simulink model "bluetooth_voice_article"  (Simulink 4.00)
settings: Solver=VariableStepDiscrete  StartTime=0.0  StopTime=2.7  RelTol=1e-3
PreLoadFcn:
  | bluetooth_init;
StopFcn:
  | ratio=sum((hops>=29) & (hops<=49))/length(hops)
values from neighbouring files (symbols this model uses):
  Access_Code = zeros(72,1); Access_Code(1:2:72)=1    [bluetooth_init.m]
  ARQ = [1]    [bluetooth_init.m]
  awgn_channel_seed = randseed(2)    [bluetooth_init.m]
  Flow_Control = [1]    [bluetooth_init.m]
  Input_Fs = 8000    [bluetooth_init.m]
  One_Zero_Payload = zeros(240,1)    [bluetooth_init.m]
  Packet_Type = [1 0 1 0]'    [bluetooth_init.m]
  Sequence = [1]    [bluetooth_init.m]
  Slave_Address = [1 0 1]'    [bluetooth_init.m]
undefined symbols (not defined in the file or in its folder): Fs, g, jet
libraries: dspsrcs3 x20, dspsigops x11, simulink3 x10, dspsigattribs x8, bluetooth_lib x5, dspmathops x4, dspbuff3 x4, dspsnks3 x4, commsink2 x3, dspmtrx3 x3, commdigbbndfm2 x3, dspindex x2
Description:
  | Bluetooth Voice Model
  | 
  | Associated Files:
  | bluetooth_init.m: Initialization
  | bluetooth_lib.mdl: Library
  | poiss_gaus_prc3.m: Poisson S-function for 802.11
  | scomdemohecgen.c: S-function C code for CRC block
  | scomdemohecgen.dll: S-function dll for CRC block
  | input.wav: Input wave file
settings Model: Creator=Stuart McGarrity  LastModifiedBy=stuartm  SaveTime=off  SaveOutput=off  OptimizeBlockIOStorage=off  BlockReductionOpt=off
settings Model: ModifiedComment=|
  | stuartm -- Fri Jul 20 12:58:27 2001 -- Version 1.201
  | Fix for R12.1. Changed CPM modulator. Replaced enable subsystems in channel with "switch case".
settings Model: ModifiedHistory=|
  | stuartm -- Fri Jul 20 12:58:27 2001 -- Version 1.201
  | Fix for R12.1. Changed CPM modulator. Replaced enable subsystems in channel with "switch case".
  | 
  | 
  | stuartm -- Sun Jul 08 13:59:13 2001 -- Version 1.172
  | Added gain mask at output of transmitter to run it off after 374 bits.
  | 
  | stuartm -- Sun Jul 08 13:53:19 2001 -- Version 1.171
  | Changed hop generator to randint block. Put zero padiing back to before transmitter.
  | 
  | 
  | Started with bluetooth_voice2. Move zero pad from input to output of transmitter. Now only transmits 374 bits
  | 
  | Added channel option

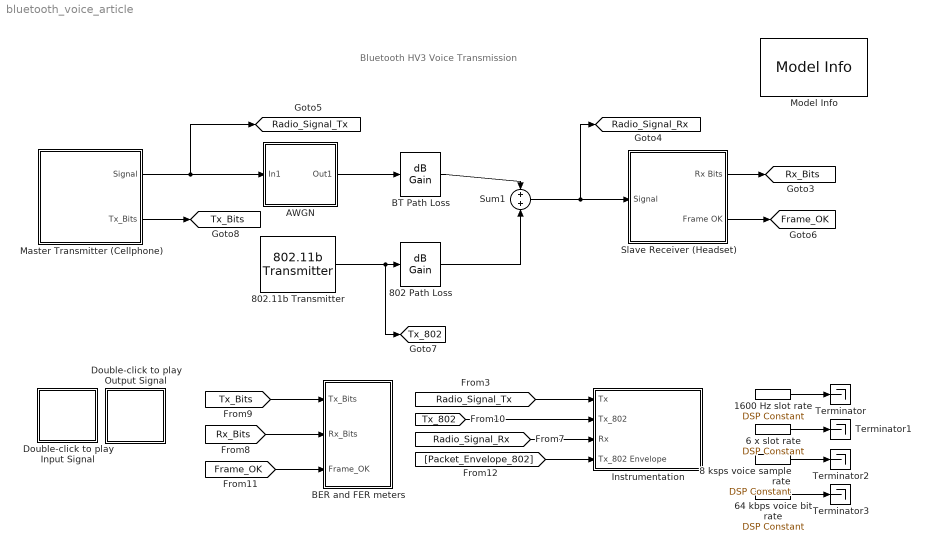
== system bluetooth_voice_article ==
  note: Bluetooth
      |  HV3 Voice Transmission
  1600 Hz slot rate : dspsrcs3/DSP Constant  Value=1  InterpretAs1D=off  SampleMode=Discrete  Ts=1/1600  FramebasedOutput=off
  6 x slot rate : dspsrcs3/DSP Constant  Value=1  InterpretAs1D=off  SampleMode=Discrete  Ts=6/1600  FramebasedOutput=off
  64 kbps voice bit rate : dspsrcs3/DSP Constant  Value=1  InterpretAs1D=off  SampleMode=Discrete  Ts=1/64000  FramebasedOutput=off
  8 ksps voice sample rate : dspsrcs3/DSP Constant  Value=1  InterpretAs1D=off  SampleMode=Discrete  Ts=1/8000  FramebasedOutput=off
  802 Path Loss : dspmathops/dB Gain  Gain=g  dB=-40  intype=Amplitude
  802.11b Transmitter : bluetooth_lib/802.11b Transmitter  On=on  rate=200  m=1e-3  v=0  power=1  Freq_Number=39  rate_seed=rate_802_seed  awgn_seed=awgn_802_seed
  AWGN : Subsystem  TreatAsAtomicUnit=on  mask(Optional channel){AWGN_On=on, EsNo=5, Power=.001, Symbol_Period=1e-6, seed=awgn_channel_seed}
      mask prompts: AWGN_On "Turn on AWGN"; EsNo "Es/No"; Power "Input Power"; Symbol_Period "Symbol Period"
      mask init:
      | if AWGN_On==1
      |    Name='On';
      | else
      |   Name='Off';
      | end;
      settings: RTWFcnNameOpts=Auto  RTWFileNameOpts=Auto
      mask Display: disp(['AWGN is ' Name])
  BER and FER meters : Subsystem
      settings: RTWFcnNameOpts=Auto  RTWFileNameOpts=Auto
  BT Path Loss : dspmathops/dB Gain  Gain=g  dB=-40  intype=Amplitude
  Double-click to play Input Signal : Subsystem  mask(Plot histogram){}
      mask init:
      | [x,y,x1,y1,x2,y2] = dspblkwao2('icon');
      settings: OpenFcn=[Input_Wave,Input_Fs]=wavread('Input.wav');sound(Input_Wave,Input_Fs);  RTWFcnNameOpts=Auto  RTWFileNameOpts=Auto
      mask Display:
      | patch(x1,y1,[1 1 1]*.5);
      | patch(x2,y2);
      | plot(x,y); plot(x1,y1)
  Double-click to play Output Signal : Subsystem  mask(Plot histogram){}
      mask init:
      | [x,y,x1,y1,x2,y2] = dspblkwao2('icon');
      settings: OpenFcn=[Output_Wave,Output_Fs]=wavread('Output.wav');sound(Output_Wave,Output_Fs);  RTWFcnNameOpts=Auto  RTWFileNameOpts=Auto
      mask Display:
      | patch(x1,y1,[1 1 1]*.5);
      | patch(x2,y2);
      | plot(x,y); plot(x1,y1)
  Instrumentation : Subsystem  TreatAsAtomicUnit=on  mask(Instrumentation){On=on, Off=off}
      mask init:
      | if strcmp(On,'on')
      |   string='Instrumentation\nis On\n(Double-Click\n to Toggle)\n ';
      |   set_param([gcb,'/State'],'Value','1');
      | else
      |   string='Instrumentation\nis Off\n(Double-Click\n to Toggle)\n ';
      |   set_param([gcb,'/State'],'Value','0');
      | end
      settings: OpenFcn=temp=get_param(gcb,'On');set_param(gcb,'On', get_param(gcb,'Off'));set_param(gcb,'Off', temp);  RTWFcnNameOpts=Auto  RTWFileNameOpts=Auto
      mask Display: disp(string);
  Master Transmitter (Cellphone) : Subsystem
      settings: RTWFcnNameOpts=Auto  RTWFileNameOpts=Auto
      mask Display: plot(0,0,100,100,[30,60,60,55,55,30,30],[10,10,90,90,70,70,10],[35,35,55,55,35],[64,45,45,64,64])
  Model Info : simulink3/Signals & Systems/Model Info  InitialBlockCM=none  BlockCM=none  Frame=on  DisplayStringWithTags=|  HorizontalTextAlignment=Center  LeftAlignmentValue=0.5  SourceBlockDiagram=bluetooth_voice  TagMaxNumber=20
      | Bluetooth Voice
      | %<ModelVersion>
  Slave Receiver (Headset) : Subsystem
      settings: RTWFcnNameOpts=Auto  RTWFileNameOpts=Auto
      mask Display: plot(15,5,95,80,[26, 28,35,44,58,85,87,92,86,59,46,46,38, 31, 27,26],[55,49,45,45,34,15,10,16,17,37,50,58,66,67,62,55],[32,34,37,42,46,46],[67,69,71,70,66,58],[27,25,24,21,23,26],[52,49,45,47,52,58],[35,38,40,42,44],[66,67,66,64,61],[34,32,38,40,34],[60,56,51,55,60])
  Sum1 : Sum  Inputs=++  SaturateOnIntegerOverflow=on
  Terminator{,1..3} (4 alike) : Terminator
  tag scope: Frame_OK=global, Radio_Signal_Rx=global, Radio_Signal_Tx=global, Rx_Bits=global, Tx_802=global, Tx_Bits=global
  wires:
  Master Transmitter (Cellphone)/1(Signal) -> [Radio_Signal_Tx], AWGN/1(In1)
  [Radio_Signal_Tx] -> Instrumentation/1(Tx)
  [Radio_Signal_Rx] -> Instrumentation/3(Rx)
  [Frame_OK] -> BER and FER meters/3(Frame_OK)
  [Tx_Bits] -> BER and FER meters/1(Tx_Bits)
  [Rx_Bits] -> BER and FER meters/2(Rx_Bits)
  [Tx_802] -> Instrumentation/2(Tx_802)
  [Packet_Envelope_802] -> Instrumentation/4(Tx_802 Envelope)
  802.11b Transmitter/1 -> [Tx_802], 802 Path Loss/1
  AWGN/1(Out1) -> BT Path Loss/1
  BT Path Loss/1 -> Sum1/1
  Sum1/1 -> [Radio_Signal_Rx], Slave Receiver (Headset)/1(Signal)
  802 Path Loss/1 -> Sum1/2
  Master Transmitter (Cellphone)/2(Tx_Bits) -> [Tx_Bits]
  Slave Receiver (Headset)/1(Rx Bits) -> [Rx_Bits]
  Slave Receiver (Headset)/2(Frame OK) -> [Frame_OK]
  1600 Hz slot rate/1 -> Terminator/1
  6 x slot rate/1 -> Terminator1/1
  8 ksps voice sample rate/1 -> Terminator2/1
  64 kbps voice bit rate/1 -> Terminator3/1

== system bluetooth_voice_article/AWGN ==
  In1 : Inport  Port=1  LatchInput=off
  Generate noise only for slot 1 : simulink3/Nonlinear/Manual Switch  sw=0  action=0
  Mode : Constant  Value=AWGN_On
  Slot 1 enable2 : dspsrcs3/Signal From Workspace  X=[1 0 0 0 0 0]  Ts=625e-6  nsamps=1  OutputAfterFinalValue=Cyclic Repetition
  Slot 1 enable3 : dspsrcs3/Signal From Workspace  X=[1 1 1 1 1 1 ]  Ts=625e-6  nsamps=1  OutputAfterFinalValue=Cyclic Repetition
  Subsystem : Subsystem  TreatAsAtomicUnit=on
      settings: RTWFcnNameOpts=Auto  RTWFileNameOpts=Auto
  Out1 : Outport  Port=1  InitialOutput=0
  wires:
  Mode/1 -> Subsystem/1(In1)
  Subsystem/1(Out1) -> Out1/1
  Slot 1 enable3/1 -> Generate noise only for slot 1/2
  Generate noise only for slot 1/1 -> Subsystem/Enable
  Slot 1 enable2/1 -> Generate noise only for slot 1/1
  In1/1 -> Subsystem/2(In2)

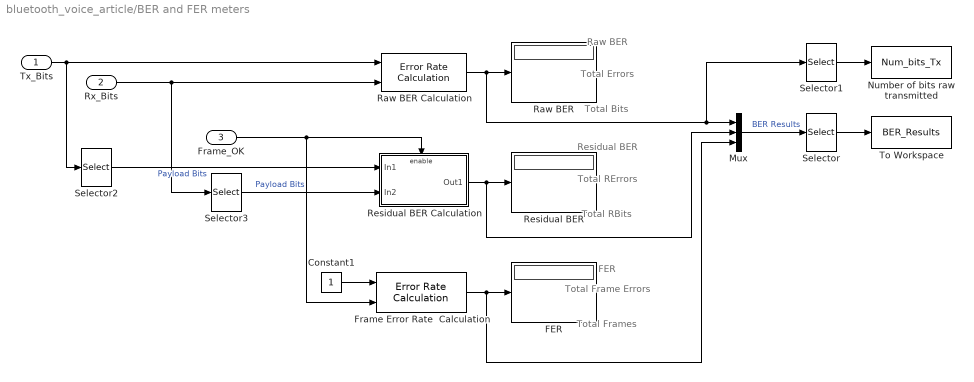
== system bluetooth_voice_article/BER and FER meters ==
  note: Residual BER
  note: Total RBits
  note: Total RErrors
  note: FER
  note: Total Frames
  note: Total Frame Errors
  note: Raw BER
  note: Total Bits
  note: Total Errors
  Tx_Bits : Inport  Port=1  LatchInput=off
  Rx_Bits : Inport  Port=2  LatchInput=off
  Frame_OK : Inport  Port=3  LatchInput=off
  Constant1 : Constant  Value=1
  FER : Display
      settings: Format=short
  Frame Error Rate  Calculation : commsink2/Error Rate Calculation  N=0  st_delay=0  cp_mode=Entire frame  subframe=[]  PMode=Port  WsName=ErrorVec  RsMode2=off  stop=off  numErr=100  maxBits=1e6
  Mux : Mux  Inputs=3
  Number of bits raw transmitted : ToWorkspace  VariableName=Num_bits_Tx  SampleTime=-1  SaveFormat=Array
      settings: MaxDataPoints=1
  Raw BER : Display
      settings: Format=short
  Raw BER Calculation : commsink2/Error Rate Calculation  N=0  st_delay=0  cp_mode=Entire frame  subframe=[]  PMode=Port  WsName=ErrorVec  RsMode2=off  stop=off  numErr=100  maxBits=1e6
  Residual BER : Display
      settings: Format=short
  Residual BER Calculation : Subsystem  TreatAsAtomicUnit=on
      settings: RTWFcnNameOpts=Auto  RTWFileNameOpts=Auto
  Selector : Selector  InputType=Vector  ElementSrc=Internal  Elements=[1 4 7]  RowSrc=Internal  Rows=1  ColumnSrc=Internal  Columns=1  InputPortWidth=9
  Selector1 : Selector  InputType=Vector  ElementSrc=Internal  Elements=[3]  RowSrc=Internal  Rows=1  ColumnSrc=Internal  Columns=1  InputPortWidth=3
  Selector2 : Selector  InputType=Vector  ElementSrc=Internal  Elements=[127:366]  RowSrc=Internal  Rows=1  ColumnSrc=Internal  Columns=1  InputPortWidth=366
  Selector3 : Selector  InputType=Vector  ElementSrc=Internal  Elements=[127:366]  RowSrc=Internal  Rows=1  ColumnSrc=Internal  Columns=1  InputPortWidth=366
  To Workspace : ToWorkspace  VariableName=BER_Results  SampleTime=-1  SaveFormat=Array
      settings: MaxDataPoints=1
  wires:
  Residual BER Calculation/1(Out1) -> Residual BER/1, Mux/2
  Frame_OK/1 -> Residual BER Calculation/Enable, Frame Error Rate  Calculation/2
  Frame Error Rate  Calculation/1 -> FER/1, Mux/3
  Tx_Bits/1 -> Raw BER Calculation/1, Selector2/1
  Rx_Bits/1 -> Raw BER Calculation/2, Selector3/1
  Raw BER Calculation/1 -> Raw BER/1, Mux/1, Selector1/1
  Mux/1 -> Selector/1  "BER Results"
  Selector/1 -> To Workspace/1
  Constant1/1 -> Frame Error Rate  Calculation/1
  Selector1/1 -> Number of bits raw transmitted/1
  Selector3/1 -> Residual BER Calculation/2(In2)  "Payload Bits"
  Selector2/1 -> Residual BER Calculation/1(In1)  "Payload Bits"

== system bluetooth_voice_article/Double-click to play Input Signal ==

== system bluetooth_voice_article/Double-click to play Output Signal ==

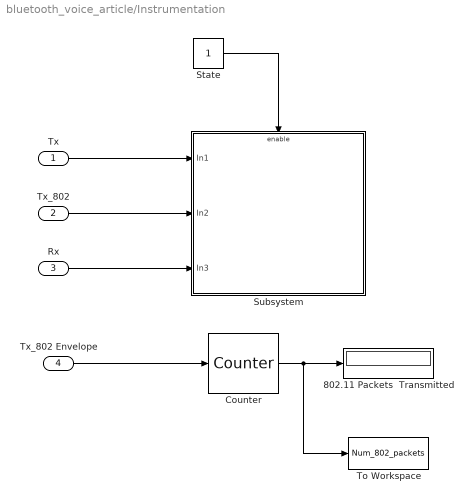
== system bluetooth_voice_article/Instrumentation ==
  Tx : Inport  Port=1  LatchInput=off
  Tx_802 : Inport  Port=2  LatchInput=off
  Rx : Inport  Port=3  LatchInput=off
  Tx_802 Envelope : Inport  Port=4  LatchInput=off
  802.11 Packets  Transmitted : Display
      settings: Format=short
  Counter : dspswit3/Counter  Direction=Up  CountEvent=Rising edge  CounterSize=User defined  MaxCount=1000  InitialCount=0  Output=Count  HitValue=32  ResetInput=off  SamplesPerFrame=1  Ts=1
  State : Constant  Value=1
  Subsystem : Subsystem  TreatAsAtomicUnit=on
      settings: RTWFcnNameOpts=Auto  RTWFileNameOpts=Auto
  To Workspace : ToWorkspace  VariableName=Num_802_packets  SampleTime=-1  SaveFormat=Array
      settings: MaxDataPoints=1
  wires:
  Rx/1 -> Subsystem/3(In3)
  Tx/1 -> Subsystem/1(In1)
  Tx_802/1 -> Subsystem/2(In2)
  Tx_802 Envelope/1 -> Counter/1
  State/1 -> Subsystem/Enable
  Counter/1 -> 802.11 Packets  Transmitted/1, To Workspace/1

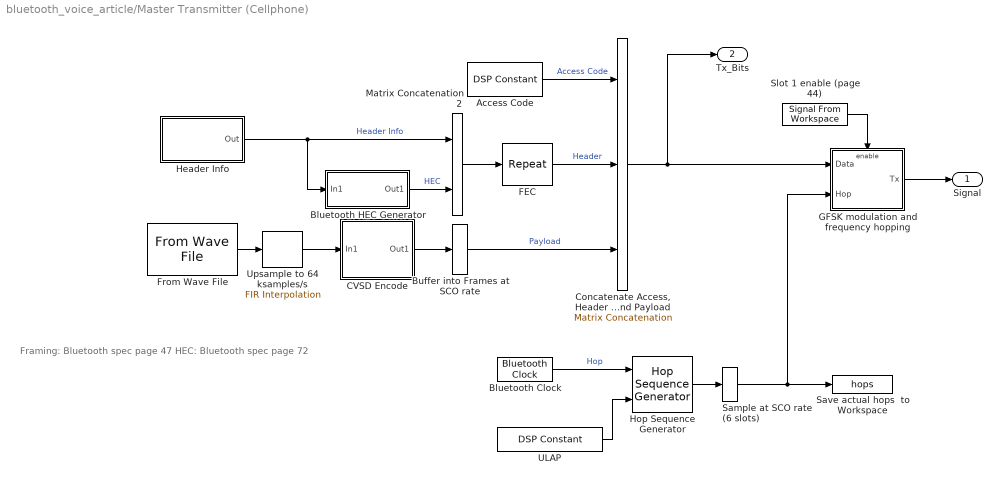
== system bluetooth_voice_article/Master Transmitter (Cellphone) ==
  note: Framing: Bluetooth spec page 47
      | HEC: Bluetooth spec page 72
  Access Code : dspsrcs3/DSP Constant  Value=Access_Code  InterpretAs1D=off  SampleMode=Discrete  Ts=30*(1/Input_Fs)  FramebasedOutput=on
  Bluetooth Clock : bluetooth_lib/Bluetooth Clock  Ts=(1/1600)/2
  Bluetooth HEC Generator : Subsystem  mask(Bluetooth HEC Generator){uap=[1 0 0 1 0 1 1 0]}
      mask help: Compute the Bluetooth Header Error Check (HEC) as specified in section 5.4 of the Bluetooth specification. The Upper Address Part (UAP) is used to initialize the state of the encoder. The UAP is an 8-bit vector, LSB first.
      settings: RTWFcnNameOpts=Auto  RTWFileNameOpts=Auto
      mask Display: disp('Bluetooth\nHEC Generator')
  Buffer into Frames at SCO rate : dspbuff3/Buffer  N=240  V=0  ic=One_Zero_Payload
  CVSD Encode : Subsystem  mask(CVSD Encoder){min_step=10, max_step=1280, accum_decay=1-1/32, step_decay=1-1/1024}
      mask prompts: min_step "Minimum Step Size"; max_step "Maximum Step Size"; accum_decay "Accumulator Decay"; step_decay "Step Decay"
      mask help: Encode a 64 K samples per sec speech signal into a 64Kbps bit stream.
      mask init:
      | pos_accum_max = 2^15 - 1;
      | neg_accum_max = -2^15 + 1;
      settings: RTWFcnNameOpts=Auto  RTWFileNameOpts=Auto
      mask Display: disp('CVSD\nEncode')
  "Concatenate Access, Header and Payload" : simulink3/Signals & Systems/Matrix Concatenation  numInports=3  catMethod=Vertical
  FEC : dspsigops/Repeat  N=3  ic=0  mode=Maintain input frame rate
  From Wave File : dspsrcs3/From Wave File  FileName=Input.wav  SamplesPerFrame=1  MinBufSize=256
  GFSK modulation and frequency hopping : Subsystem  TreatAsAtomicUnit=on
      settings: RTWFcnNameOpts=Auto  RTWFileNameOpts=Auto
  Header Info : Subsystem
      settings: RTWFcnNameOpts=Auto  RTWFileNameOpts=Auto
      mask Display: disp('Header Info')
  Hop Sequence Generator : bluetooth_lib/Hop Sequence Generator  Hop_Mode=Connection State Hop Sequence  hop_seed=hop_seed  fixed_hop_freq=fixed_hop_freq
  Matrix Concatenation2 : simulink3/Signals & Systems/Matrix Concatenation  numInports=2  catMethod=Vertical
  Sample at SCO rate (6 slots) : ZeroOrderHold  SampleTime=6*625e-6
  Save actual hops  to Workspace : ToWorkspace  VariableName=hops  SampleTime=-1  SaveFormat=Array
  Slot 1 enable (page 44) : dspsrcs3/Signal From Workspace  X=[1 0 0 0 0 0]  Ts=625e-6  nsamps=1  OutputAfterFinalValue=Cyclic Repetition
  ULAP : dspsrcs3/DSP Constant  Value=hex2dec('2a96ef25')  InterpretAs1D=off  SampleMode=Discrete  Ts=(1/1600)/2  FramebasedOutput=off
  Upsample to 64 ksamples/s : dspmlti3/FIR Interpolation  h=interp_coeffs  L=8  framing=Maintain input frame size  outputBufInitCond=0
  Signal : Outport  Port=1
  Tx_Bits : Outport  Port=2
  wires:
  Slot 1 enable (page 44)/1 -> GFSK modulation and frequency hopping/Enable
  GFSK modulation and frequency hopping/1(Tx) -> Signal/1
  CVSD Encode/1(Out1) -> Buffer into Frames at SCO rate/1
  From Wave File/1 -> Upsample to 64 ksamples/s/1
  Upsample to 64 ksamples/s/1 -> CVSD Encode/1(In1)
  Buffer into Frames at SCO rate/1 -> "Concatenate Access, Header and Payload"/3  "Payload"
  Access Code/1 -> "Concatenate Access, Header and Payload"/1  "Access Code"
  "Concatenate Access, Header and Payload"/1 -> Tx_Bits/1, GFSK modulation and frequency hopping/1(Data)
  FEC/1 -> "Concatenate Access, Header and Payload"/2  "Header"
  Header Info/1(Out) -> Bluetooth HEC Generator/1(In1), Matrix Concatenation2/1  "Header Info"
  Bluetooth HEC Generator/1(Out1) -> Matrix Concatenation2/2  "HEC"
  Matrix Concatenation2/1 -> FEC/1
  Hop Sequence Generator/1 -> Sample at SCO rate (6 slots)/1
  ULAP/1 -> Hop Sequence Generator/2
  Sample at SCO rate (6 slots)/1 -> GFSK modulation and frequency hopping/2(Hop), Save actual hops  to Workspace/1
  Bluetooth Clock/1 -> Hop Sequence Generator/1  "Hop"

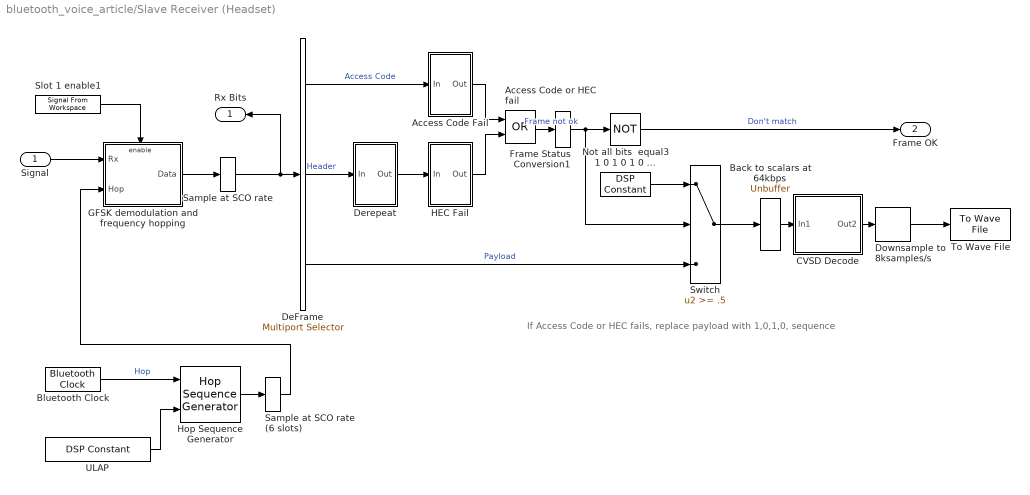
== system bluetooth_voice_article/Slave Receiver (Headset) ==
  note: If Access Code or HEC fails,
      | replace payload with 1,0,1,0, sequence
  Signal : Inport  Port=1  LatchInput=off
  1 0 1 0 1 0 ... : dspsrcs3/DSP Constant  Value=One_Zero_Payload  InterpretAs1D=off  SampleMode=Discrete  Ts=30*(1/Input_Fs)  FramebasedOutput=on
  Access Code Fail : Subsystem
      settings: RTWFcnNameOpts=Auto  RTWFileNameOpts=Auto
  Access Code or HEC fail : Logic  Operator=OR  Inputs=2
  Back to scalars at 64kbps : dspbuff3/Unbuffer  ic=0
  Bluetooth Clock : bluetooth_lib/Bluetooth Clock  Ts=(1/1600)/2
  CVSD Decode : Subsystem  TreatAsAtomicUnit=on  mask(CVSD Decoder){min_step=10, max_step=1280, accum_decay=1-1/32, step_decay=1-1/1024}
      mask prompts: min_step "Minimum Step Size"; max_step "Maximum Step Size"; accum_decay "Accumulator Decay"; step_decay "Step Decay"
      mask init:
      | pos_accum_max = 2^15 - 1;
      | neg_accum_max = -2^15 + 1;
      settings: RTWFcnNameOpts=Auto  RTWFileNameOpts=Auto
      mask Display: disp('CVSD\nDecoder')
  DeFrame : dspindex/Multiport Selector  rowsOrCols=Rows  idxCellArray={ 1:72, 73:126,127:366}  idxErrMode=Clip Index
  Derepeat : Subsystem
      settings: RTWFcnNameOpts=Auto  RTWFileNameOpts=Auto
  Downsample to 8ksamples/s : dspsigops/Downsample  N=8  phase=0  ic=0  smode=Allow multirate  fmode=Maintain input frame size
  Frame Status Conversion1 : dspsigattribs/Frame Status Conversion  growRefPort=off  outframe=Sample-based
  GFSK demodulation and frequency hopping : Subsystem  TreatAsAtomicUnit=on
      settings: RTWFcnNameOpts=Auto  RTWFileNameOpts=Auto
  HEC Fail : Subsystem
      settings: RTWFcnNameOpts=Auto  RTWFileNameOpts=Auto
  Hop Sequence Generator : bluetooth_lib/Hop Sequence Generator  Hop_Mode=Connection State Hop Sequence  hop_seed=hop_seed  fixed_hop_freq=fixed_hop_freq
  Not all bits  equal3 : Logic  Operator=NOT  Inputs=1
  Sample at SCO rate : ZeroOrderHold  SampleTime=6*625e-6
  Sample at SCO rate (6 slots) : ZeroOrderHold  SampleTime=6*625e-6
  Slot 1 enable1 : dspsrcs3/Signal From Workspace  X=[1 0 0 0 0 0]  Ts=625e-6  nsamps=1  OutputAfterFinalValue=Cyclic Repetition
  Switch : Switch  Threshold=.5
  To Wave File : dspsnks3/To Wave File  filename=Output  sampleWidth=8  MinNumSamples=256
  ULAP : dspsrcs3/DSP Constant  Value=hex2dec('2a96ef25')  InterpretAs1D=off  SampleMode=Discrete  Ts=(1/1600)/2  FramebasedOutput=off
  Rx Bits : Outport  Orientation=left  Port=1
  Frame OK : Outport  Port=2
  wires:
  GFSK demodulation and frequency hopping/1(Data) -> Sample at SCO rate/1
  Slot 1 enable1/1 -> GFSK demodulation and frequency hopping/Enable
  Signal/1 -> GFSK demodulation and frequency hopping/1(Rx)
  Not all bits  equal3/1 -> Frame OK/1  "Don't match"
  CVSD Decode/1(Out2) -> Downsample to 8ksamples/s/1
  Downsample to 8ksamples/s/1 -> To Wave File/1
  Back to scalars at 64kbps/1 -> CVSD Decode/1(In1)
  Sample at SCO rate/1 -> DeFrame/1, Rx Bits/1
  Sample at SCO rate (6 slots)/1 -> GFSK demodulation and frequency hopping/2(Hop)
  DeFrame/2 -> Derepeat/1(In)  "Header"
  DeFrame/3 -> Switch/3  "Payload"
  DeFrame/1 -> Access Code Fail/1(In)  "Access Code"
  Access Code or HEC fail/1 -> Frame Status Conversion1/1  "Frame not ok"
  1 0 1 0 1 0 .../1 -> Switch/1
  Access Code Fail/1(Out) -> Access Code or HEC fail/1
  Derepeat/1(Out) -> HEC Fail/1(In)
  HEC Fail/1(Out) -> Access Code or HEC fail/2
  Frame Status Conversion1/1 -> Switch/2, Not all bits  equal3/1
  Switch/1 -> Back to scalars at 64kbps/1
  Hop Sequence Generator/1 -> Sample at SCO rate (6 slots)/1
  ULAP/1 -> Hop Sequence Generator/2
  Bluetooth Clock/1 -> Hop Sequence Generator/1  "Hop"

== system bluetooth_voice_article/AWGN/Subsystem ==
  In1 : Inport  Port=1  LatchInput=off
  In2 : Inport  Port=2  LatchInput=off
  Enable : EnablePort
  Add noise : Subsystem  TreatAsAtomicUnit=on
      settings: RTWFcnNameOpts=Auto  RTWFileNameOpts=Auto
  If : If  NumInputs=1  IfExpression=u1 == 0  ShowElse=on
  Merge : Merge  Inputs=2  AllowUnequalInputPortWidths=off  InputPortOffsets=[]
  Pass Through : Subsystem  TreatAsAtomicUnit=on
      settings: RTWFcnNameOpts=Auto  RTWFileNameOpts=Auto
  Out1 : Outport  Port=1
  wires:
  Add noise/1(Out1) -> Merge/2
  Pass Through/1(Out1) -> Merge/1
  If/1 -> Pass Through/Action
  In2/1 -> Pass Through/1(In1), Add noise/1(In1)
  If/2 -> Add noise/Action
  In1/1 -> If/1
  Merge/1 -> Out1/1

== system bluetooth_voice_article/BER and FER meters/Residual BER Calculation ==
  In1 : Inport  Port=1  LatchInput=off
  In2 : Inport  Port=2  LatchInput=off
  Enable : EnablePort
  Error Rate Calculation : commsink2/Error Rate Calculation  N=0  st_delay=0  cp_mode=Entire frame  subframe=[]  PMode=Port  WsName=ErrorVec  RsMode2=off  stop=off  numErr=100  maxBits=1e6
  Out1 : Outport  Port=1
  wires:
  In1/1 -> Error Rate Calculation/1
  Error Rate Calculation/1 -> Out1/1
  In2/1 -> Error Rate Calculation/2

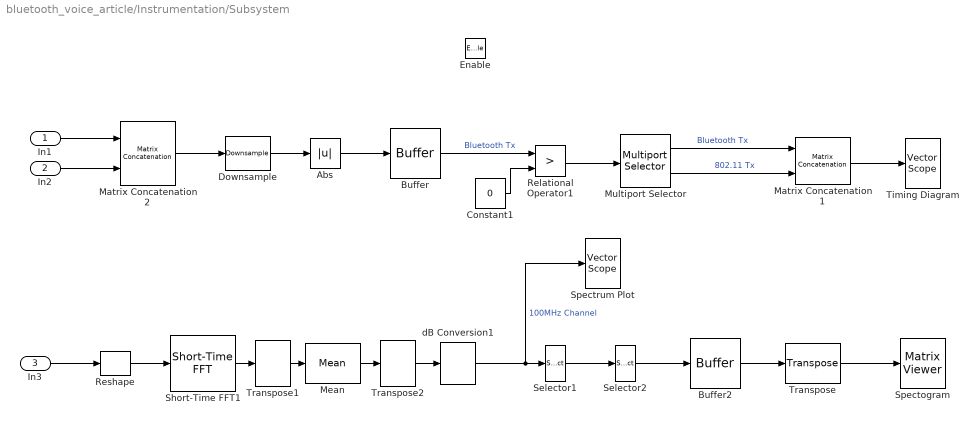
== system bluetooth_voice_article/Instrumentation/Subsystem ==
  In1 : Inport  Port=1  LatchInput=off
  In2 : Inport  Port=2  LatchInput=off
  In3 : Inport  Port=3  LatchInput=off
  Enable : EnablePort
  Abs : Abs  SaturateOnIntegerOverflow=on
  Buffer : dspbuff3/Buffer  N=60*500  V=59*500  ic=0
  Buffer2 : dspbuff3/Buffer  N=60  V=59  ic=-70
  Constant1 : Constant  Value=0
  Downsample : dspsigops/Downsample  N=125  phase=0  ic=0  smode=Allow multirate  fmode=Maintain input frame rate
  Matrix Concatenation1 : simulink3/Signals & Systems/Matrix Concatenation  numInports=2  catMethod=Horizontal
  Matrix Concatenation2 : simulink3/Signals & Systems/Matrix Concatenation  numInports=2  catMethod=Horizontal
  Mean : dspstat3/Mean  run=off  reset_popup=None
  Multiport Selector : dspindex/Multiport Selector  rowsOrCols=Columns  idxCellArray={ 1,2}  idxErrMode=Clip Index
  Relational Operator1 : RelationalOperator  Operator=>
  Reshape : simulink3/Signals & Systems/Reshape  OutputDimensionality=Customize  OutputDimensions=[500,125]
  Selector1 : Selector  InputType=Vector  ElementSrc=Internal  Elements=[257:512 1:256]  RowSrc=Internal  Rows=1  ColumnSrc=Internal  Columns=1  InputPortWidth=512
  Selector2 : Selector  InputType=Vector  ElementSrc=Internal  Elements=7:506  RowSrc=Internal  Rows=1  ColumnSrc=Internal  Columns=1  InputPortWidth=512
  Short-Time FFT1 : dspspect3/Short-Time FFT  wintype=Hanning  Rs=50  beta=5  winsamp=Periodic  inheritFFT=off  fftsize=512  navg=1
  Spectogram : dspsnks3/Matrix Viewer  ImageParams=on  CMapStr=jet(256)  AxisColorbar=on  AxisParams=on  AxisOrigin=Lower left corner  XLabel=Time Index  YLabel=Frequency Index  ZLabel=dB Magnitude  FigPos=[65 269 688 127]  AxisZoom=on
      settings: YMin=-60  YMax=-30
  Spectrum Plot : dspsnks3/Vector Scope  ScopeProperties=on  Domain=Frequency  HorizSpan=1  DisplayProperties=off  AxisGrid=on  Memory=off  FrameNumber=on  AxisLegend=on  AxisZoom=off  OpenScopeAtSimStart=on  OpenScopeImmediately=off  FigPos=[2 605 774 120]  AxisProperties=off  XUnits=Hertz  XRange=[-Fs/2...Fs/2]  InheritXIncr=off  XIncr=1e-8  XLabel=Time  YUnits=Magnitude  YLabel=Magnitude, dB  LineProperties=off  LineStyles=--
      settings: YMin=-80.906815143504  YMax=-25.7732682054945
  Timing Diagram : dspsnks3/Vector Scope  ScopeProperties=on  Domain=User-defined  HorizSpan=1  DisplayProperties=off  AxisGrid=on  Memory=off  FrameNumber=on  AxisLegend=on  AxisZoom=off  OpenScopeAtSimStart=on  OpenScopeImmediately=off  FigPos=[8 427 776 129]  AxisProperties=off  XUnits=Hertz  XRange=[0...Fs/2]  InheritXIncr=off  XIncr=125*1e-8  XLabel=Time (s)  YUnits=dB  YLabel=Amplitude  LineProperties=off  LineStyles=-|-  LineColors=[0 1 0]|[1 0 0]
      settings: YMin=0  YMax=1.1
  Transpose : dspmtrx3/Transpose  Hermitian=off
  Transpose1 : dspmtrx3/Transpose  Hermitian=off
  Transpose2 : dspmtrx3/Transpose  Hermitian=off
  dB Conversion1 : dspmathops/dB Conversion  dBtype=dB  intype=Power  R=1  fuzz=on
  wires:
  Transpose/1 -> Spectogram/1
  Buffer2/1 -> Transpose/1
  Abs/1 -> Buffer/1
  Downsample/1 -> Abs/1
  dB Conversion1/1 -> Selector1/1, Spectrum Plot/1  "100MHz Channel"
  Short-Time FFT1/1 -> Transpose1/1
  Selector1/1 -> Selector2/1
  Selector2/1 -> Buffer2/1
  Matrix Concatenation1/1 -> Timing Diagram/1
  In3/1 -> Reshape/1
  Reshape/1 -> Short-Time FFT1/1
  Mean/1 -> Transpose2/1
  Transpose1/1 -> Mean/1
  Transpose2/1 -> dB Conversion1/1
  Constant1/1 -> Relational Operator1/2
  Buffer/1 -> Relational Operator1/1  "Bluetooth Tx"
  In2/1 -> Matrix Concatenation2/2
  In1/1 -> Matrix Concatenation2/1
  Matrix Concatenation2/1 -> Downsample/1
  Relational Operator1/1 -> Multiport Selector/1
  Multiport Selector/1 -> Matrix Concatenation1/1  "Bluetooth Tx"
  Multiport Selector/2 -> Matrix Concatenation1/2  "802.11 Tx"

== system bluetooth_voice_article/Master Transmitter (Cellphone)/Bluetooth HEC Generator ==
  In1 : Inport  Port=1  LatchInput=off
  Frame Status Conversion : dspsigattribs/Frame Status Conversion  growRefPort=off  outframe=Sample-based
  Frame Status Conversion1 : dspsigattribs/Frame Status Conversion  growRefPort=on  outframe=Sample-based
  S-Function Builder : S-Function  AncestorBlock=|  FunctionName=scomdemohecgen  Parameters=uap  PortCounts=[]  SFunctionModules=scomdemohecgen_wrapper  WizardData=DataTag0
      | simulink3/Functions
      | & Tables/Basic S-Function
      | Builder
      mask init:
      | val = [[.9  0.75 0.75 1 1 .9 .9 1]',[1 1 0.75 0.75 .9 .9 1 .9]'];
      | sys = get_param(gcb,'FunctionName');
      settings: CopyFcn=set_param(gcb,'LinkStatus','none')  OpenFcn=sfunctionwizard(gcbh)
      mask Display:
      | plot(val(:,1),val(:,2))
      | disp(sys)
  Out1 : Outport  Port=1
  wires:
  Frame Status Conversion/1 -> S-Function Builder/1
  Frame Status Conversion1/1 -> Out1/1
  In1/1 -> Frame Status Conversion1/2, Frame Status Conversion/1
  S-Function Builder/1 -> Frame Status Conversion1/1

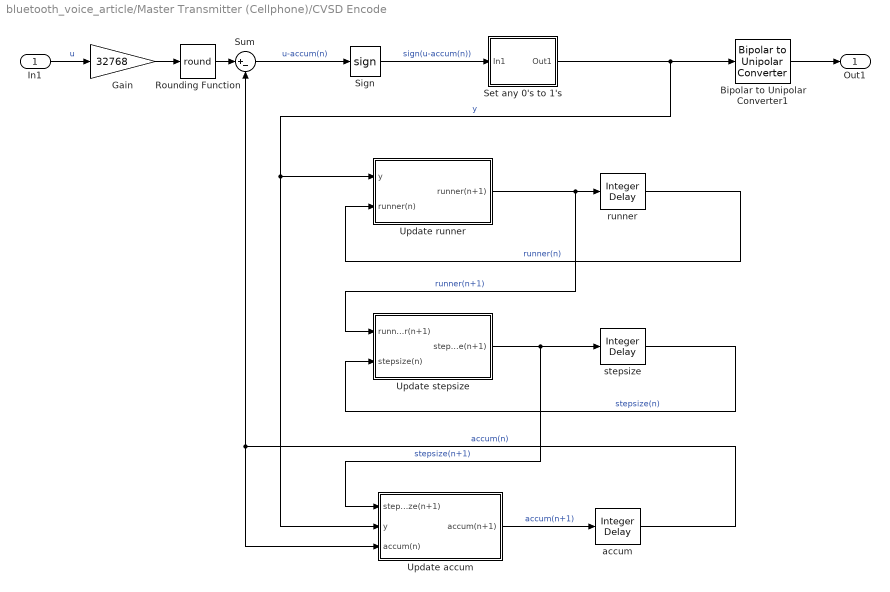
== system bluetooth_voice_article/Master Transmitter (Cellphone)/CVSD Encode ==
  In1 : Inport  Port=1  LatchInput=off
  Bipolar to Unipolar Converter1 : commutil2/Bipolar to Unipolar Converter  M=2  polarity=Negative
  Gain : Gain  Gain=32768  Multiplication=Element-wise(K.*u)  SaturateOnIntegerOverflow=on
  Rounding Function : Rounding  Operator=round
  Set any 0's to 1's : Subsystem
      settings: RTWFcnNameOpts=Auto  RTWFileNameOpts=Auto
  Sign : Signum
  Sum : Sum  Inputs=|+-  SaturateOnIntegerOverflow=on
  Update accum : Subsystem
      settings: RTWFcnNameOpts=Auto  RTWFileNameOpts=Auto
  Update runner : Subsystem
      settings: RTWFcnNameOpts=Auto  RTWFileNameOpts=Auto
  Update stepsize : Subsystem
      settings: RTWFcnNameOpts=Auto  RTWFileNameOpts=Auto
  accum : dspsigops/Integer Delay  delay=1  ic=0
  runner : dspsigops/Integer Delay  delay=1  ic=10
  stepsize : dspsigops/Integer Delay  delay=1  ic=min_step
  Out1 : Outport  Port=1
  wires:
  Gain/1 -> Rounding Function/1
  Rounding Function/1 -> Sum/1
  Bipolar to Unipolar Converter1/1 -> Out1/1
  In1/1 -> Gain/1  "u"
  Sum/1 -> Sign/1  "u-accum(n)"
  accum/1 -> Sum/2, Update accum/3(accum(n))  "accum(n)"
  Set any 0's to 1's/1(Out1) -> Bipolar to Unipolar Converter1/1, Update runner/1(y), Update accum/2(y)  "y"
  runner/1 -> Update runner/2(runner(n))  "runner(n)"
  Update runner/1(runner(n+1)) -> runner/1, Update stepsize/1(runner(n+1))  "runner(n+1)"
  Sign/1 -> Set any 0's to 1's/1(In1)  "sign(u-accum(n))"
  stepsize/1 -> Update stepsize/2(stepsize(n))  "stepsize(n)"
  Update stepsize/1(stepsize(n+1)) -> stepsize/1, Update accum/1(stepsize(n+1))  "stepsize(n+1)"
  Update accum/1(accum(n+1)) -> accum/1  "accum(n+1)"

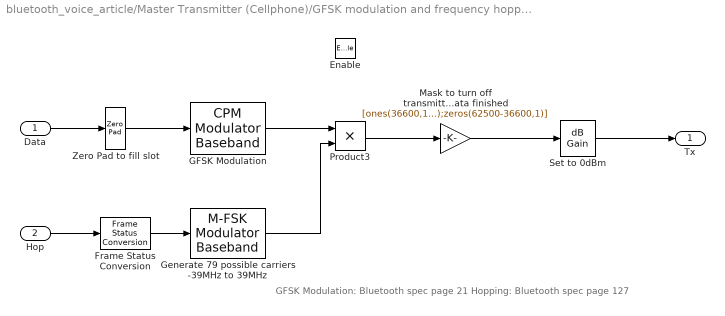
== system bluetooth_voice_article/Master Transmitter (Cellphone)/GFSK modulation and frequency hopping ==
  note: GFSK Modulation: Bluetooth spec page 21
      | Hopping: Bluetooth spec page 127
  Data : Inport  Port=1  LatchInput=off  SampleTime=625e-6
  Hop : Inport  Port=2  LatchInput=off  SampleTime=625e-6
  Enable : EnablePort
  Frame Status Conversion : dspsigattribs/Frame Status Conversion  growRefPort=off  outframe=Frame-based
  GFSK Modulation : commdigbbndcpm2/CPM Modulator Baseband  Mnum=2  inputType=Bit  mappingType=Binary  modIdx=0.32  pulseShape=Gaussian  BT=0.5  rollOff=0.2  pulseLength=1  preHistory=1  phaseOffset=0  samplesPerSymbol=100
  "Generate 79 possible carriers -39MHz to 39MHz " : commdigbbndfm2/M-FSK Modulator Baseband  M=79  InType=Integer  Enc=Binary  freqSep=1e6  phaseType=Continuous  numSamp=6.25e4
  Mask to turn off transmitter after data finished : Gain  Gain=[ones(36600,1);zeros(62500-36600,1)]  Multiplication=Element-wise(K.*u)  SaturateOnIntegerOverflow=on
  Product3 : Product  Inputs=2  Multiplication=Element-wise(.*)  SaturateOnIntegerOverflow=on
  Set to 0dBm : dspmathops/dB Gain  Gain=g  dB=-20  intype=Amplitude
  Zero Pad to fill slot : dspsigops/Zero Pad  zpadAlong=Columns  numOutRows=625  numOutCols=1  trunc_flag=None
  Tx : Outport  Port=1  OutputWhenDisabled=reset  InitialOutput=0
  wires:
  Data/1 -> Zero Pad to fill slot/1
  Hop/1 -> Frame Status Conversion/1
  GFSK Modulation/1 -> Product3/1
  Product3/1 -> Mask to turn off transmitter after data finished/1
  "Generate 79 possible carriers -39MHz to 39MHz "/1 -> Product3/2
  Mask to turn off transmitter after data finished/1 -> Set to 0dBm/1
  Set to 0dBm/1 -> Tx/1
  Frame Status Conversion/1 -> "Generate 79 possible carriers -39MHz to 39MHz "/1
  Zero Pad to fill slot/1 -> GFSK Modulation/1

== system bluetooth_voice_article/Master Transmitter (Cellphone)/Header Info ==
  Header3 : dspsrcs3/DSP Constant  Value=Slave_Address  InterpretAs1D=off  SampleMode=Discrete  Ts=30*(1/Input_Fs)  FramebasedOutput=on
  Header4 : dspsrcs3/DSP Constant  Value=Packet_Type  InterpretAs1D=off  SampleMode=Discrete  Ts=30*(1/Input_Fs)  FramebasedOutput=on
  Header5 : dspsrcs3/DSP Constant  Value=Flow_Control  InterpretAs1D=off  SampleMode=Discrete  Ts=30*(1/Input_Fs)  FramebasedOutput=on
  Header6 : dspsrcs3/DSP Constant  Value=ARQ  InterpretAs1D=off  SampleMode=Discrete  Ts=30*(1/Input_Fs)  FramebasedOutput=on
  Header7 : dspsrcs3/DSP Constant  Value=Sequence  InterpretAs1D=off  SampleMode=Discrete  Ts=30*(1/Input_Fs)  FramebasedOutput=on
  Matrix Concatenation1 : simulink3/Signals & Systems/Matrix Concatenation  numInports=5  catMethod=Vertical
  Out : Outport  Port=1
  wires:
  Header3/1 -> Matrix Concatenation1/1  "Slave address"
  Header4/1 -> Matrix Concatenation1/2  "Packet type"
  Header5/1 -> Matrix Concatenation1/3  "Flow control"
  Header6/1 -> Matrix Concatenation1/4  "ARQ"
  Header7/1 -> Matrix Concatenation1/5  "Sequence"
  Matrix Concatenation1/1 -> Out/1  "Header Info"

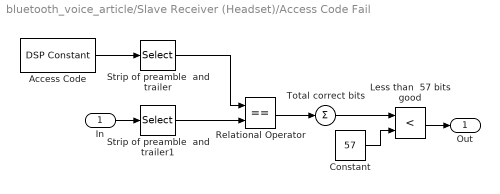
== system bluetooth_voice_article/Slave Receiver (Headset)/Access Code Fail ==
  In : Inport  Port=1  LatchInput=off
  Access Code : dspsrcs3/DSP Constant  Value=Access_Code  InterpretAs1D=off  SampleMode=Discrete  Ts=30*(1/Input_Fs)  FramebasedOutput=on
  Constant : Constant  Value=57
  Less than  57 bits good : RelationalOperator  Operator=<
  Relational Operator : RelationalOperator  Operator===
  Strip of preamble  and trailer : Selector  InputType=Vector  ElementSrc=Internal  Elements=[5:68]  RowSrc=Internal  Rows=1  ColumnSrc=Internal  Columns=1  InputPortWidth=72
  Strip of preamble  and trailer1 : Selector  InputType=Vector  ElementSrc=Internal  Elements=[5:68]  RowSrc=Internal  Rows=1  ColumnSrc=Internal  Columns=1  InputPortWidth=72
  Total correct bits : Sum  Inputs=1  SaturateOnIntegerOverflow=on
  Out : Outport  Port=1
  wires:
  Access Code/1 -> Strip of preamble  and trailer/1
  Relational Operator/1 -> Total correct bits/1
  Strip of preamble  and trailer1/1 -> Relational Operator/2
  Strip of preamble  and trailer/1 -> Relational Operator/1
  Total correct bits/1 -> Less than  57 bits good/1
  Constant/1 -> Less than  57 bits good/2
  In/1 -> Strip of preamble  and trailer1/1
  Less than  57 bits good/1 -> Out/1

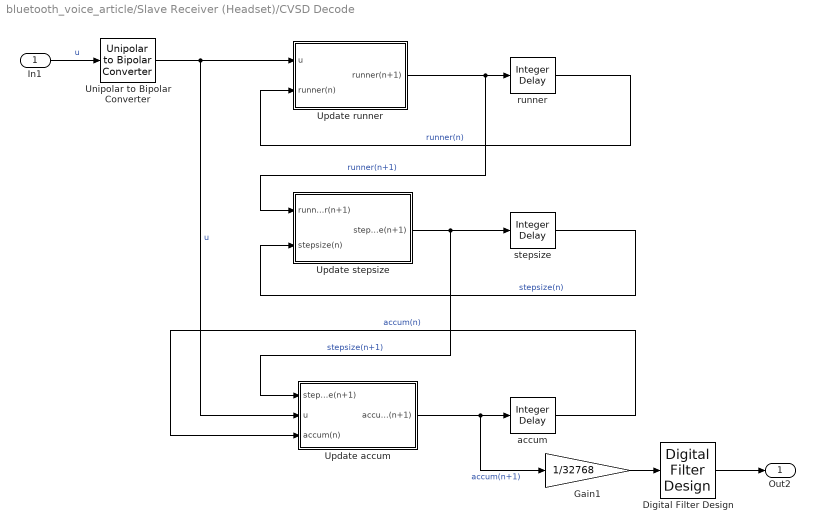
== system bluetooth_voice_article/Slave Receiver (Headset)/CVSD Decode ==
  In1 : Inport  Port=1  LatchInput=off
  Digital Filter Design : dsparch3/Digital Filter Design
  Gain1 : Gain  Gain=1/32768  Multiplication=Element-wise(K.*u)  SaturateOnIntegerOverflow=on
  Unipolar to Bipolar Converter : commutil2/Unipolar to Bipolar Converter  M=2  polarity=Negative
  Update accum : Subsystem
      settings: RTWFcnNameOpts=Auto  RTWFileNameOpts=Auto
  Update runner : Subsystem
      settings: RTWFcnNameOpts=Auto  RTWFileNameOpts=Auto
  Update stepsize : Subsystem
      settings: RTWFcnNameOpts=Auto  RTWFileNameOpts=Auto
  accum : dspsigops/Integer Delay  delay=1  ic=0
  runner : dspsigops/Integer Delay  delay=1  ic=10
  stepsize : dspsigops/Integer Delay  delay=1  ic=min_step
  Out2 : Outport  Port=1
  wires:
  In1/1 -> Unipolar to Bipolar Converter/1  "u"
  accum/1 -> Update accum/3(accum(n))  "accum(n)"
  runner/1 -> Update runner/2(runner(n))  "runner(n)"
  Update runner/1(runner(n+1)) -> runner/1, Update stepsize/1(runner(n+1))  "runner(n+1)"
  stepsize/1 -> Update stepsize/2(stepsize(n))  "stepsize(n)"
  Update stepsize/1(stepsize(n+1)) -> stepsize/1, Update accum/1(stepsize(n+1))  "stepsize(n+1)"
  Update accum/1(accum(n+1)) -> accum/1, Gain1/1  "accum(n+1)"
  Unipolar to Bipolar Converter/1 -> Update accum/2(u), Update runner/1(u)  "u"
  Digital Filter Design/1 -> Out2/1
  Gain1/1 -> Digital Filter Design/1

== system bluetooth_voice_article/Slave Receiver (Headset)/Derepeat ==
  In : Inport  Port=1  LatchInput=off
  Constant1 : Constant  Value=.5
  Decode FEC : commsequence2/Derepeat  N=3  ic=0  mode=Maintain input frame rate
  Threshold : RelationalOperator  Operator=>
  Out : Outport  Port=1
  wires:
  Constant1/1 -> Threshold/2
  Decode FEC/1 -> Threshold/1
  In/1 -> Decode FEC/1
  Threshold/1 -> Out/1  "HEC"

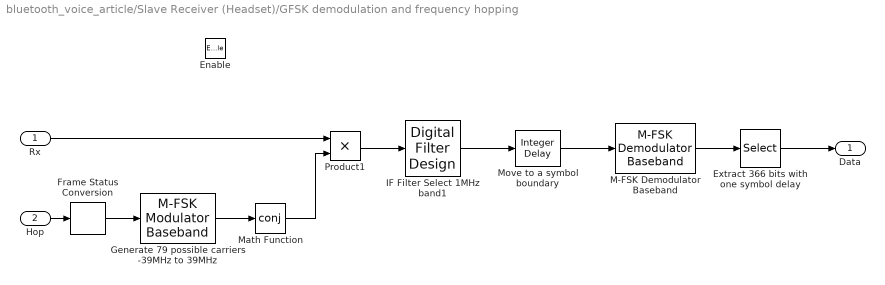
== system bluetooth_voice_article/Slave Receiver (Headset)/GFSK demodulation and frequency hopping ==
  Rx : Inport  Port=1  LatchInput=off
  Hop : Inport  Port=2  LatchInput=off  SampleTime=625e-6
  Enable : EnablePort
  Extract 366 bits with one symbol delay : Selector  InputType=Vector  ElementSrc=Internal  Elements=[2:367]  RowSrc=Internal  Rows=1  ColumnSrc=Internal  Columns=1  InputPortWidth=625
  Frame Status Conversion : dspsigattribs/Frame Status Conversion  growRefPort=off  outframe=Frame-based
  "Generate 79 possible carriers -39MHz to 39MHz " : commdigbbndfm2/M-FSK Modulator Baseband  M=79  InType=Integer  Enc=Binary  freqSep=1e6  phaseType=Continuous  numSamp=6.25e4
  IF Filter Select 1MHz band1 : dsparch3/Digital Filter Design
  M-FSK Demodulator Baseband : commdigbbndfm2/M-FSK Demodulator Baseband  M=2  OutType=Bit  Dec=Binary  freqSep=2*150e3  numSamp=100
  Math Function : Math  Operator=conj  OutputSignalType=auto
  Move to a symbol boundary : dspsigops/Integer Delay  delay=100-45  ic=0
  Product1 : Product  Inputs=2  Multiplication=Element-wise(.*)  SaturateOnIntegerOverflow=on
  Data : Outport  Port=1  OutputWhenDisabled=reset  InitialOutput=0
  wires:
  M-FSK Demodulator Baseband/1 -> Extract 366 bits with one symbol delay/1
  Rx/1 -> Product1/1
  Product1/1 -> IF Filter Select 1MHz band1/1
  Hop/1 -> Frame Status Conversion/1
  Math Function/1 -> Product1/2
  "Generate 79 possible carriers -39MHz to 39MHz "/1 -> Math Function/1
  Frame Status Conversion/1 -> "Generate 79 possible carriers -39MHz to 39MHz "/1
  Extract 366 bits with one symbol delay/1 -> Data/1
  IF Filter Select 1MHz band1/1 -> Move to a symbol boundary/1
  Move to a symbol boundary/1 -> M-FSK Demodulator Baseband/1

== system bluetooth_voice_article/Slave Receiver (Headset)/HEC Fail ==
  In : Inport  Port=1  LatchInput=off
  Any HEC bits not matching : Logic  Operator=OR  Inputs=1
  Bluetooth HEC Generator1 : Subsystem  mask(Bluetooth HEC Generator){uap=[1 0 0 1 0 1 1 0]}
      mask help: Compute the Bluetooth Header Error Check (HEC) as specified in section 5.4 of the Bluetooth specification. The Upper Address Part (UAP) is used to initialize the state of the encoder. The UAP is an 8-bit vector, LSB first.
      settings: RTWFcnNameOpts=Auto  RTWFileNameOpts=Auto
      mask Display: disp('Bluetooth\nHEC Generator')
  Demux : Demux  Outputs=[10 8]  BusSelectionMode=off
  Relational Operator1 : RelationalOperator  Operator=~=
  Out : Outport  Port=1
  wires:
  Relational Operator1/1 -> Any HEC bits not matching/1
  Demux/1 -> Bluetooth HEC Generator1/1(In1)
  Demux/2 -> Relational Operator1/2
  Bluetooth HEC Generator1/1(Out1) -> Relational Operator1/1
  In/1 -> Demux/1
  Any HEC bits not matching/1 -> Out/1

== system bluetooth_voice_article/AWGN/Subsystem/Add noise ==
  In1 : Inport  Port=1  LatchInput=off
  Action Port : ActionPort  InitializeStates=held  ActionType=else
  AWGN Channel1 : commchan2/AWGN Channel  seed=seed  noiseMode="Signal to noise ratio  (Es/No)"  EsNodB=EsNo  SNRdB=10  Ps=Power  Tsym=Symbol_Period  variance=1
  Contiguous Copy : dspsigattribs/Contiguous Copy
  Out1 : Outport  Port=1
  wires:
  In1/1 -> AWGN Channel1/1
  Contiguous Copy/1 -> Out1/1
  AWGN Channel1/1 -> Contiguous Copy/1

== system bluetooth_voice_article/AWGN/Subsystem/Pass Through ==
  In1 : Inport  Port=1  LatchInput=off
  Action Port : ActionPort  InitializeStates=held  ActionType=then
  Out1 : Outport  Port=1
  wires:
  In1/1 -> Out1/1

== system bluetooth_voice_article/Master Transmitter (Cellphone)/CVSD Encode/Set any 0's to 1's ==
  In1 : Inport  Port=1  LatchInput=off
  If : If  NumInputs=1  IfExpression=u1 ==0  ShowElse=on
  Merge : Merge  Inputs=2  AllowUnequalInputPortWidths=off  InputPortOffsets=[]
  Pass through : Subsystem  TreatAsAtomicUnit=on
      settings: RTWFcnNameOpts=Auto  RTWFileNameOpts=Auto
  Set to 1 : Subsystem  TreatAsAtomicUnit=on
      settings: RTWFcnNameOpts=Auto  RTWFileNameOpts=Auto
  Out1 : Outport  Port=1
  wires:
  If/1 -> Set to 1/Action
  In1/1 -> Pass through/1(In1), If/1
  If/2 -> Pass through/Action
  Set to 1/1(1) -> Merge/1
  Pass through/1(Out1=In1) -> Merge/2
  Merge/1 -> Out1/1  "y"

== system bluetooth_voice_article/Master Transmitter (Cellphone)/CVSD Encode/Update accum ==
  stepsize(n+1) : Inport  Port=1  LatchInput=off
  y : Inport  Port=2  LatchInput=off
  accum(n) : Inport  Port=3  LatchInput=off
  Gain : Gain  Gain=accum_decay  Multiplication=Element-wise(K.*u)  SaturateOnIntegerOverflow=on
  Product : Product  Inputs=2  Multiplication=Element-wise(.*)  SaturateOnIntegerOverflow=on
  Saturation : Saturate  UpperLimit=pos_accum_max  LowerLimit=neg_accum_max  LinearizeAsGain=on
  Sum1 : Sum  Inputs=|++  SaturateOnIntegerOverflow=on
  accum(n+1) : Outport  Port=1
  wires:
  Gain/1 -> Saturation/1
  Product/1 -> Sum1/1  "y*stepsize"
  Sum1/1 -> Gain/1
  stepsize(n+1)/1 -> Product/1
  y/1 -> Product/2
  accum(n)/1 -> Sum1/2
  Saturation/1 -> accum(n+1)/1

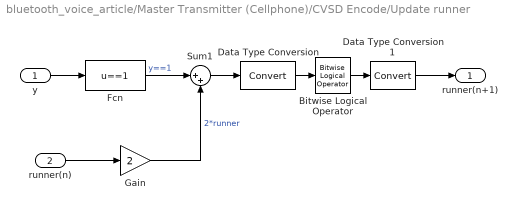
== system bluetooth_voice_article/Master Transmitter (Cellphone)/CVSD Encode/Update runner ==
  y : Inport  Port=1  LatchInput=off
  runner(n) : Inport  Port=2  LatchInput=off
  Bitwise Logical Operator : simulink3/Math/Bitwise Logical Operator  Operator=AND  Operand2=15
  Data Type Conversion : DataTypeConversion  DataType=uint16  SaturateOnIntegerOverflow=on
  Data Type Conversion1 : DataTypeConversion  DataType=double  SaturateOnIntegerOverflow=on
  Fcn : Fcn  Expr=u==1
  Gain : Gain  Gain=2  Multiplication=Element-wise(K.*u)  SaturateOnIntegerOverflow=on
  Sum1 : Sum  Inputs=|++  SaturateOnIntegerOverflow=on
  runner(n+1) : Outport  Port=1
  wires:
  Gain/1 -> Sum1/2  "2*runner"
  Fcn/1 -> Sum1/1  "y==1"
  Sum1/1 -> Data Type Conversion/1
  Data Type Conversion/1 -> Bitwise Logical Operator/1
  y/1 -> Fcn/1
  Bitwise Logical Operator/1 -> Data Type Conversion1/1
  runner(n)/1 -> Gain/1
  Data Type Conversion1/1 -> runner(n+1)/1

== system bluetooth_voice_article/Master Transmitter (Cellphone)/CVSD Encode/Update stepsize ==
  runner(n+1) : Inport  Port=1  LatchInput=off
  stepsize(n) : Inport  Port=2  LatchInput=off
  If : If  NumInputs=1  IfExpression=(u1 == 0) | (u1== 15)  ShowElse=on
  Merge1 : Merge  Inputs=2  AllowUnequalInputPortWidths=off  InputPortOffsets=[]
  Update : Subsystem  TreatAsAtomicUnit=on
      settings: RTWFcnNameOpts=Auto  RTWFileNameOpts=Auto
  Update1 : Subsystem  TreatAsAtomicUnit=on
      settings: RTWFcnNameOpts=Auto  RTWFileNameOpts=Auto
  stepsize(n+1) : Outport  Port=1
  wires:
  If/2 -> Update1/Action
  If/1 -> Update/Action  "(runner == 0) | (runner == 15)"
  Update/1(stepsize(n+1)) -> Merge1/1
  stepsize(n)/1 -> Update1/1(stepsize), Update/1(stepsize)
  Update1/1(stepsize(n+1)) -> Merge1/2
  runner(n+1)/1 -> If/1
  Merge1/1 -> stepsize(n+1)/1

== system bluetooth_voice_article/Slave Receiver (Headset)/CVSD Decode/Update accum ==
  stepsize(n+1) : Inport  Port=1  LatchInput=off
  u : Inport  Port=2  LatchInput=off
  accum(n) : Inport  Port=3  LatchInput=off
  Gain : Gain  Gain=accum_decay  Multiplication=Element-wise(K.*u)  SaturateOnIntegerOverflow=on
  Product : Product  Inputs=2  Multiplication=Element-wise(.*)  SaturateOnIntegerOverflow=on
  Saturation : Saturate  UpperLimit=pos_accum_max  LowerLimit=neg_accum_max  LinearizeAsGain=on
  Sum1 : Sum  Inputs=|++  SaturateOnIntegerOverflow=on
  accum(n+1) : Outport  Port=1
  wires:
  Product/1 -> Sum1/1  "y*stepsize"
  Sum1/1 -> Gain/1
  stepsize(n+1)/1 -> Product/1
  u/1 -> Product/2
  accum(n)/1 -> Sum1/2
  Gain/1 -> Saturation/1
  Saturation/1 -> accum(n+1)/1

== system bluetooth_voice_article/Slave Receiver (Headset)/CVSD Decode/Update runner ==
  u : Inport  Port=1  LatchInput=off
  runner(n) : Inport  Port=2  LatchInput=off
  Bitwise Logical Operator : simulink3/Math/Bitwise Logical Operator  Operator=AND  Operand2=15
  Data Type Conversion : DataTypeConversion  DataType=uint16  SaturateOnIntegerOverflow=on
  Data Type Conversion1 : DataTypeConversion  DataType=double  SaturateOnIntegerOverflow=on
  Fcn : Fcn  Expr=u==1
  Gain : Gain  Gain=2  Multiplication=Element-wise(K.*u)  SaturateOnIntegerOverflow=on
  Sum1 : Sum  Inputs=|++  SaturateOnIntegerOverflow=on
  runner(n+1) : Outport  Port=1
  wires:
  Gain/1 -> Sum1/2  "2*runner"
  Fcn/1 -> Sum1/1  "y==1"
  Sum1/1 -> Data Type Conversion/1
  Data Type Conversion/1 -> Bitwise Logical Operator/1
  u/1 -> Fcn/1
  Bitwise Logical Operator/1 -> Data Type Conversion1/1
  runner(n)/1 -> Gain/1
  Data Type Conversion1/1 -> runner(n+1)/1

== system bluetooth_voice_article/Slave Receiver (Headset)/CVSD Decode/Update stepsize ==
  runner(n+1) : Inport  Port=1  LatchInput=off
  stepsize(n) : Inport  Port=2  LatchInput=off
  If : If  NumInputs=1  IfExpression=(u1 == 0) | (u1== 15)  ShowElse=on
  Merge1 : Merge  Inputs=2  AllowUnequalInputPortWidths=off  InputPortOffsets=[]
  Update : Subsystem  TreatAsAtomicUnit=on
      settings: RTWFcnNameOpts=Auto  RTWFileNameOpts=Auto
  Update1 : Subsystem  TreatAsAtomicUnit=on
      settings: RTWFcnNameOpts=Auto  RTWFileNameOpts=Auto
  stepsize(n+1) : Outport  Port=1
  wires:
  If/1 -> Update/Action  "(runner == 0) | (runner == 15)"
  Update/1(stepsize(n+1)) -> Merge1/1
  stepsize(n)/1 -> Update1/1(stepsize), Update/1(stepsize)
  If/2 -> Update1/Action
  Update1/1(stepsize(n+1)) -> Merge1/2
  runner(n+1)/1 -> If/1
  Merge1/1 -> stepsize(n+1)/1

== system bluetooth_voice_article/Slave Receiver (Headset)/HEC Fail/Bluetooth HEC Generator1 ==
  In1 : Inport  Port=1  LatchInput=off
  Frame Status Conversion : dspsigattribs/Frame Status Conversion  growRefPort=off  outframe=Sample-based
  Frame Status Conversion1 : dspsigattribs/Frame Status Conversion  growRefPort=on  outframe=Sample-based
  S-Function Builder : S-Function  AncestorBlock=|  FunctionName=scomdemohecgen  Parameters=uap  PortCounts=[]  SFunctionModules=scomdemohecgen_wrapper
      | simulink3/Functions
      | & Tables/Basic S-Function
      | Builder
      mask init:
      | val = [[.9  0.75 0.75 1 1 .9 .9 1]',[1 1 0.75 0.75 .9 .9 1 .9]'];
      | sys = get_param(gcb,'FunctionName');
      settings: CopyFcn=set_param(gcb,'LinkStatus','none')  OpenFcn=sfunctionwizard(gcbh)
      mask Display:
      | plot(val(:,1),val(:,2))
      | disp(sys)
  Out1 : Outport  Port=1
  wires:
  Frame Status Conversion/1 -> S-Function Builder/1
  Frame Status Conversion1/1 -> Out1/1
  In1/1 -> Frame Status Conversion1/2, Frame Status Conversion/1
  S-Function Builder/1 -> Frame Status Conversion1/1

== system bluetooth_voice_article/Master Transmitter (Cellphone)/CVSD Encode/Set any 0's to 1's/Pass through ==
  In1 : Inport  Port=1  LatchInput=off
  Action Port : ActionPort  InitializeStates=held  ActionType=else
  Out1=In1 : Outport  Port=1
  wires:
  In1/1 -> Out1=In1/1

== system bluetooth_voice_article/Master Transmitter (Cellphone)/CVSD Encode/Set any 0's to 1's/Set to 1 ==
  Action Port : ActionPort  InitializeStates=held  ActionType=then
  DSP Constant : dspsrcs3/DSP Constant  Value=1  InterpretAs1D=on  SampleMode=Discrete  Ts=1/64000  FramebasedOutput=off
  1 : Outport  Port=1
  wires:
  DSP Constant/1 -> 1/1

== system bluetooth_voice_article/Master Transmitter (Cellphone)/CVSD Encode/Update stepsize/Update ==
  stepsize : Inport  Port=1  LatchInput=off
  Action Port : ActionPort  InitializeStates=held  ActionType=then
  Constant : Constant  Value=min_step
  Constant1 : Constant  Value=max_step
  MinMax : MinMax  Function=min  Inputs=2
  Sum2 : Sum  Inputs=|++  SaturateOnIntegerOverflow=on
  stepsize(n+1) : Outport  Port=1
  wires:
  Constant/1 -> Sum2/1
  Sum2/1 -> MinMax/1
  Constant1/1 -> MinMax/2
  MinMax/1 -> stepsize(n+1)/1
  stepsize/1 -> Sum2/2

== system bluetooth_voice_article/Master Transmitter (Cellphone)/CVSD Encode/Update stepsize/Update1 ==
  stepsize : Inport  Port=1  LatchInput=off
  Action Port : ActionPort  InitializeStates=held  ActionType=else
  Constant1 : Constant  Value=min_step
  Gain : Gain  Gain=step_decay  Multiplication=Element-wise(K.*u)  SaturateOnIntegerOverflow=on
  MinMax : MinMax  Function=max  Inputs=2
  stepsize(n+1) : Outport  Port=1
  wires:
  MinMax/1 -> stepsize(n+1)/1
  Constant1/1 -> MinMax/2
  Gain/1 -> MinMax/1
  stepsize/1 -> Gain/1

== system bluetooth_voice_article/Slave Receiver (Headset)/CVSD Decode/Update stepsize/Update ==
  stepsize : Inport  Port=1  LatchInput=off
  Action Port : ActionPort  InitializeStates=held  ActionType=then
  Constant : Constant  Value=min_step
  Constant1 : Constant  Value=max_step
  MinMax : MinMax  Function=min  Inputs=2
  Sum2 : Sum  Inputs=|++  SaturateOnIntegerOverflow=on
  stepsize(n+1) : Outport  Port=1
  wires:
  Constant/1 -> Sum2/1
  Sum2/1 -> MinMax/1
  Constant1/1 -> MinMax/2
  MinMax/1 -> stepsize(n+1)/1
  stepsize/1 -> Sum2/2

== system bluetooth_voice_article/Slave Receiver (Headset)/CVSD Decode/Update stepsize/Update1 ==
  stepsize : Inport  Port=1  LatchInput=off
  Action Port : ActionPort  InitializeStates=held  ActionType=else
  Constant1 : Constant  Value=min_step
  Gain : Gain  Gain=step_decay  Multiplication=Element-wise(K.*u)  SaturateOnIntegerOverflow=on
  MinMax : MinMax  Function=max  Inputs=2
  stepsize(n+1) : Outport  Port=1
  wires:
  MinMax/1 -> stepsize(n+1)/1
  Constant1/1 -> MinMax/2
  Gain/1 -> MinMax/1
  stepsize/1 -> Gain/1
